simulink library "xblocks_library_downconverter"  (Simulink 7.6)
settings: Solver=ode45  SolverMode=SingleTasking  StartTime=0.0  StopTime=10.0  RelTol=1e-3
libraries: xbsIndex_r4 x104
settings Model: Creator=mdexter  LastModifiedBy=chenhong

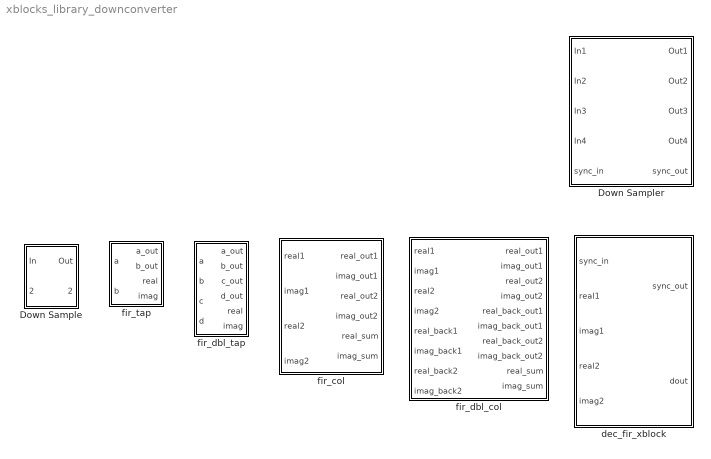
== system xblocks_library_downconverter ==
  Down Sample : Subsystem  mask(Down Sample){dec_rate=4, input_clk_period=1, input_period=2, xilinx=off, ext_en=off}
      mask prompts: dec_rate "Rate Change"; input_clk_period "Actual Input Clock Period"; input_period "Effective Input Sampling Period"; xilinx "Use Xilinx Down Sample?"; ext_en "External enable port?"
      mask help: Down Sample by using a periodically enabled register
      mask init:
      | config.source=str2func('downsample_init_xblock');
      | config.depend=get_dependlist('downsample');
      | config.toplevel=gcb;
      | set_param(gcb,'LinkStatus','inactive');
      | xBlock(config, {config.toplevel,...
      |     'dec_rate', dec_rate, ...
      |     'input_clk_period', input_clk_period, ...
      |     'input_period', input_period, ...
      |     'xilinx', xilinx, ...
      |     'ext_en', ext_en});
      settings: AttributesFormatString=|
      | Rate change: 4
      | clock(actualy/effective): 1/2
  Down Sampler : Subsystem  mask(Parallel Downconverter (xBlock)){n_inputs=4, dec_rate=3, xilinx=off, input_clk_rate=0}
      mask prompts: n_inputs "number of inputs"; dec_rate "Decimation rate"; xilinx "Use Xilinx version of Down Sample?"; input_clk_rate "Input Clock Rate"
      mask help: Parallely downconvert.
      mask init:
      | config.source=str2func('parallel_downsampler_init_xblock');
      | config.depend=get_dependlist('parallel_downsampler');
      | config.toplevel=gcb;
      | set_param(gcb,'LinkStatus','inactive');
      | xBlock(config, {config.toplevel,...
      |     'n_inputs', n_inputs, ...
      |     'dec_rate', dec_rate, ...
      |     'xilinx', xilinx, ...
      |     'input_clk_rate', input_clk_rate});
      settings: AttributesFormatString=Decimation Rate = 3
  dec_fir_xblock : Subsystem  mask(dec_fir (xBlock)){n_inputs=2, coeff=[1 2 3 4], n_bits=4, quantization=Truncate, add_latency=1, mult_latency=2, coeff_bit_width=25, coeff_bin_pt=24, adder_tree_hdl=off}
      mask prompts: n_inputs "Number of Parallel Streams"; coeff "Coefficients"; n_bits "Bit Width Out"; quantization "Quantization Behavior"; add_latency "Add Latency"; mult_latency "Mult Latency"; coeff_bit_width "Coefficient bit width"; coeff_bin_pt "Coefficient binary point"; adder_tree_hdl "Implement first stage of adder trees after multiplication as behavioural HDL"
      mask help:
      | FIR filter which can handle multiple time samples in parallel and decimates down to 1 time sample.  If coefficients are symmetric, will automatically fold before multiplying.
      | (xBlock version)
      mask init:
      | config.source=str2func('dec_fir_init_xblock');
      | config.toplevel=gcb;
      | config.depend = get_dependlist('dec_fir');
      | set_param(gcb,'LinkStatus','inactive');
      | xBlock(config, ...
      |         {config.toplevel,n_inputs,coeff,n_bits,quantization,add_latency,...
      |          mult_latency, coeff_bit_width,coeff_bin_pt,adder_tree_hdl});
      settings: AttributesFormatString=|
      | 4 taps
      | 4_3 r/i
      mask StyleString: edit,edit,edit,popup(Truncate|Round  (unbiased: +/- Inf)|Round  (unbiased: Even Values)),edit,edit,edit,edit,checkbox
      mask CallbackString:
      | coeff = (get_param(gcb,'coeff'));
      | n_inputs = (get_param(gcb,'n_inputs'));
      | if ~isempty(coeff) && ~isempty(n_inputs)
      |     coeff = eval(coeff);
      |     n_inputs = eval(n_inputs);
      |     coeff_round = round(coeff*1e16)*1e-16;
      |     if mod(length(coeff)/n_inputs,1) ~=0
      |         errordlg('The number of coefficients must be integer multiples of the number of inputs');
      |         set_param(gcb,'n_inputs','');
      |     end
      |     num_fir_col = length(coeff)/n_inputs;
      |     if coeff_round(1:int32(length(coeff)/2)) == coeff_round(length(coeff):-1:int32(length(coeff)/2)+1)
      |         num_fir_col = num_fir_col / 2;
      |     end
      |     if num_fir_col <= 0
      |         errordlg(['error: the number of column must be a positive integer. num_fir_col = ', num2str(num_fir_col)]);
      |         set_param(gcb,'n_inputs','');
      |     end
      | end
      | |coeff = (get_param(gcb,'coeff'));
      | n_inputs = (get_param(gcb,'n_inputs'));
      | if ~isempty(coeff) && ~isempty(n_inputs)
      |     coeff = eval(coeff);
      |     n_inputs = eval(n_inputs);
      |     coeff_round = round(coeff*1e16)*1e-16;
      |     if mod(length(coeff)/n_inputs,1) ~=0
      |         errordlg('The number of coefficients must be integer multiples of the number of inputs');
      |         set_param(gcb,'coeff','');
      |     end
      |     num_fir_col = length(coeff)/n_inputs;
      |     if coeff_round(1:int32(length(coeff)/2)) == coeff_round(length(coeff):-1:int32(length(coeff)/2)+1)
      |         num_fir_col = num_fir_col / 2;
      |     end
      |     if num_fir_col <= 0
      |         errordlg(['error: the number of column must be a positive integer. num_fir_col = ', num2str(num_fir_col)]);
      |         set_param(gcb,'coeff','');
      |     end
      | end
      | |||||||
  fir_col : Subsystem  mask(fir_col){n_inputs=2, coeff=[2 3], add_latency=1, mult_latency=2, coeff_bit_width=25, coeff_bin_pt=24, adder_tree_hdl=off}
      mask prompts: n_inputs "Inputs"; coeff "Coefficients"; add_latency "Add latency"; mult_latency "Mult Latency"; coeff_bit_width "Coefficient bit width"; coeff_bin_pt "Coefficient binary point"; adder_tree_hdl "Implement first stage of adder trees on output as behavioural HDL"
      mask help: (xBlock version)
      mask init:
      | config.source = str2func('fir_col_init_xblock');
      | config.toplevel = gcb;
      | config.depend = get_dependlist('fir_col');
      | set_param(gcb,'LinkStatus','inactive');
      | xBlock(config, {config.toplevel, ...
      |     n_inputs,...
      |     coeff, ...
      |     add_latency, ...
      |     mult_latency, ...
      |     coeff_bit_width, ...
      |     coeff_bin_pt, ...
      |     adder_tree_hdl});
      mask Help: eval('xlWeb(''http://casper.berkeley.edu/wiki/Fir_col'')')
  fir_dbl_col : Subsystem  mask(fir_dbl_col){n_inputs=2, coeff=[0.1 0.2 0.3 0.4], add_latency=1, mult_latency=2, coeff_bit_width=25, coeff_bin_pt=24, adder_tree_hdl=off}
      mask prompts: n_inputs "Inputs"; coeff "Coefficients"; add_latency "Add latency"; mult_latency "Mult Latency"; coeff_bit_width "Coefficient bit width"; coeff_bin_pt "Coefficient binary point"; adder_tree_hdl "Implement first stage of adder trees on output as behavioural HDL"
      mask help: (xBlock version)
      mask init:
      | config.source = str2func('fir_dbl_col_init_xblock');
      | config.toplevel = gcb;
      | config.depend = get_dependlist('fir_dbl_col');
      | set_param(gcb,'LinkStatus','inactive');
      | xBlock(config, {config.toplevel, ...
      |      n_inputs, ...
      |      coeff, ...
      |      add_latency, ...
      |      mult_latency, ...
      |      coeff_bit_width, ...
      |      coeff_bin_pt,  ...
      |      adder_tree_hdl});
      mask Help: eval('xlWeb(''http://casper.berkeley.edu/wiki/Fir_dbl_col'')')
  fir_dbl_tap : Subsystem  mask(fir_dbl_tap){factor=0.073384, add_latency=1, mult_latency=2, coeff_bit_width=18, coeff_bin_pt=17}
      mask prompts: add_latency "Add latency"; mult_latency "Mult latency"; coeff_bit_width "Coefficient bit width"; coeff_bin_pt "Coefficient binary point"
      mask help: (xBlock version)
      mask init:
      | config.source = str2func('fir_dbl_tap_init_xblock');
      | config.toplevel = gcb;
      | config.depend = get_dependlist('fir_dbl_tap');
      | set_param(gcb,'LinkStatus','inactive');
      | xBlock(config, {config.toplevel, ...
      |     factor, ...
      |     add_latency, ...
      |     mult_latency, ...
      |     coeff_bit_width, ...
      |     coeff_bin_pt});
      mask Help: eval('xlWeb(''http://casper.berkeley.edu/wiki/Fir_dbl_tap'')')
  fir_tap : Subsystem  mask(fir_tap){factor=1, latency=2, coeff_bit_width=25, coeff_bin_pt=24}
      mask prompts: latency "Mult latency"; coeff_bit_width "Coefficient bit width"; coeff_bin_pt "Coefficient binary point"
      mask help:
      | Multiplies input data with factor specified.
      | (xBlock version)
      mask init:
      | config.source = str2func('fir_tap_init_xblock');
      | config.toplevel = gcb;
      | config.depend = get_dependlist('fir_tap');
      | set_param(gcb,'LinkStatus','inactive');
      | xBlock(config,{config.toplevel, ...
      |     factor, ...
      |     latency, ...
      |     coeff_bit_width, ...
      |     coeff_bin_pt});
      mask Help: eval('xlWeb(''http://casper.berkeley.edu/wiki/Fir_tap'')')

== system xblocks_library_downconverter/Down Sample ==
  In : Inport
  sync_in : Inport  Port=2
  Register : xbsIndex_r4/Register  init=0  rst=off  en=on  dbl_ovrd=off  block_type=register
  en_gen : Subsystem
      settings: AttributesFormatString=|
      | hold period: 8
      | explicit clk period:on , input clk period:1
  sync_delay : xbsIndex_r4/Delay  rst=off  infoeditControl=Selection of Reset will increase slice count due to use of real FFs and instead of SRLs  en=off  latency=1  dbl_ovrd=off  reg_retiming=off  block_type=delay
  Out : Outport
  sync_out : Outport  Port=2
  wires:
  sync_in/1 -> sync_delay/1, en_gen/1(sync_in)
  sync_delay/1 -> sync_out/1
  Register/1 -> Out/1
  en_gen/1(en_out) -> Register/2  "en"
  In/1 -> Register/1

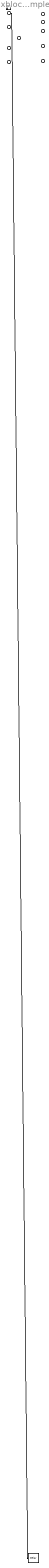
== system xblocks_library_downconverter/Down Sampler ==
  In1 : Inport
  In2 : Inport  Port=2
  In3 : Inport  Port=3
  In4 : Inport  Port=4
  sync_in : Inport  Port=5
  Down_sample1 : Subsystem
  delay1 : xbsIndex_r4/Delay  rst=off  infoeditControl=Selection of Reset will increase slice count due to use of real FFs and instead of SRLs  en=off  latency=2  dbl_ovrd=off  reg_retiming=off  block_type=delay
  Out1 : Outport
  Out2 : Outport  Port=2
  Out3 : Outport  Port=3
  Out4 : Outport  Port=4
  sync_out : Outport  Port=5
  wires:
  In1/1 -> delay1/1

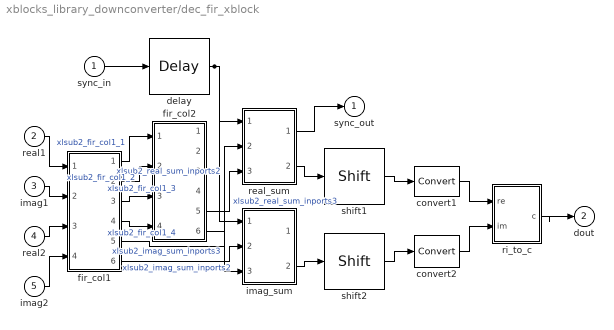
== system xblocks_library_downconverter/dec_fir_xblock ==
  sync_in : Inport
  real1 : Inport  Port=2
  imag1 : Inport  Port=3
  real2 : Inport  Port=4
  imag2 : Inport  Port=5
  convert1 : xbsIndex_r4/Convert  gui_display_data_type=Fixed-point  arith_type="Signed  (2's comp)"  n_bits=4  bin_pt=3  float_type=Single  exp_bits=8  fraction_bits=24  quantization=Truncate  overflow=Wrap  en=off  latency=1  dbl_ovrd=off  pipeline=off  block_type=convert
  convert2 : xbsIndex_r4/Convert  gui_display_data_type=Fixed-point  arith_type="Signed  (2's comp)"  n_bits=4  bin_pt=3  float_type=Single  exp_bits=8  fraction_bits=24  quantization=Truncate  overflow=Wrap  en=off  latency=1  dbl_ovrd=off  pipeline=off  block_type=convert
  delay : xbsIndex_r4/Delay  rst=off  infoeditControl=Selection of Reset will increase slice count due to use of real FFs and instead of SRLs  en=off  latency=4  dbl_ovrd=off  reg_retiming=off  block_type=delay
  fir_col1 : Subsystem
  fir_col2 : Subsystem
  imag_sum : Subsystem
      settings: AttributesFormatString=latency 1
  real_sum : Subsystem
      settings: AttributesFormatString=latency 1
  ri_to_c : Subsystem
  shift1 : xbsIndex_r4/Shift  shift_dir=Left  shift_bits=1  en=off  latency=0  precision=Full  arith_type="Signed  (2's comp)"  n_bits=16  bin_pt=14  quantization=Truncate  overflow=Wrap  dbl_ovrd=off  block_type=shift
  shift2 : xbsIndex_r4/Shift  shift_dir=Left  shift_bits=1  en=off  latency=0  precision=Full  arith_type="Signed  (2's comp)"  n_bits=16  bin_pt=14  quantization=Truncate  overflow=Wrap  dbl_ovrd=off  block_type=shift
  sync_out : Outport
  dout : Outport  Port=2
  wires:
  delay/1 -> real_sum/1(sync), imag_sum/1(sync)
  shift2/1 -> convert2/1
  imag_sum/2(dout) -> shift2/1
  shift1/1 -> convert1/1
  real_sum/2(dout) -> shift1/1
  ri_to_c/1(c) -> dout/1
  convert2/1 -> ri_to_c/2(im)
  convert1/1 -> ri_to_c/1(re)
  real_sum/1(sync_out) -> sync_out/1
  fir_col2/5(real_sum) -> real_sum/3(din2)  "xlsub2_real_sum_inports3"
  fir_col1/5(real_sum) -> real_sum/2(din1)  "xlsub2_real_sum_inports2"
  fir_col2/6(imag_sum) -> imag_sum/3(din2)  "xlsub2_imag_sum_inports3"
  fir_col1/6(imag_sum) -> imag_sum/2(din1)  "xlsub2_imag_sum_inports2"
  fir_col1/4(imag_out2) -> fir_col2/4(imag2)  "xlsub2_fir_col1_4"
  fir_col1/3(real_out2) -> fir_col2/3(real2)  "xlsub2_fir_col1_3"
  fir_col1/2(imag_out1) -> fir_col2/2(imag1)  "xlsub2_fir_col1_2"
  fir_col1/1(real_out1) -> fir_col2/1(real1)  "xlsub2_fir_col1_1"
  imag2/1 -> fir_col1/4(imag2)
  real2/1 -> fir_col1/3(real2)
  imag1/1 -> fir_col1/2(imag1)
  real1/1 -> fir_col1/1(real1)
  sync_in/1 -> delay/1

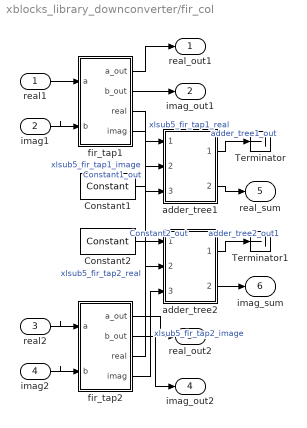
== system xblocks_library_downconverter/fir_col ==
  real1 : Inport
  imag1 : Inport  Port=2
  real2 : Inport  Port=3
  imag2 : Inport  Port=4
  Constant1 : xbsIndex_r4/Constant  arith_type=Signed (2's comp)  const=1  n_bits=16  bin_pt=14  explicit_period=on  period=1  equ=P=C  opselect=C  inp2=PCIN>>17  opr=+  inp1=P  carry=CIN  dbl_ovrd=off  block_type=constant
      settings: block_version=11.4
  Constant2 : xbsIndex_r4/Constant  arith_type=Signed (2's comp)  const=1  n_bits=16  bin_pt=14  explicit_period=on  period=1  equ=P=C  opselect=C  inp2=PCIN>>17  opr=+  inp1=P  carry=CIN  dbl_ovrd=off  block_type=constant
      settings: block_version=11.4
  Terminator : Terminator
  Terminator1 : Terminator
  adder_tree1 : Subsystem
      settings: AttributesFormatString=latency 1
  adder_tree2 : Subsystem
      settings: AttributesFormatString=latency 1
  fir_tap1 : Subsystem
  fir_tap2 : Subsystem
  real_out1 : Outport
  imag_out1 : Outport  Port=2
  real_out2 : Outport  Port=3
  imag_out2 : Outport  Port=4
  real_sum : Outport  Port=5
  imag_sum : Outport  Port=6
  wires:
  adder_tree2/1(sync_out) -> Terminator1/1  "adder_tree2_out1"
  adder_tree1/1(sync_out) -> Terminator/1  "adder_tree1_out"
  adder_tree2/2(dout) -> imag_sum/1
  fir_tap2/4(imag) -> adder_tree2/3(din2)  "xlsub5_fir_tap2_image"
  fir_tap1/4(imag) -> adder_tree2/2(din1)  "xlsub5_fir_tap1_image"
  Constant2/1 -> adder_tree2/1(sync)  "Constant2_out"
  adder_tree1/2(dout) -> real_sum/1
  fir_tap2/3(real) -> adder_tree1/3(din2)  "xlsub5_fir_tap2_real"
  fir_tap1/3(real) -> adder_tree1/2(din1)  "xlsub5_fir_tap1_real"
  Constant1/1 -> adder_tree1/1(sync)  "Constant1_out"
  fir_tap2/2(b_out) -> imag_out2/1
  fir_tap2/1(a_out) -> real_out2/1
  imag2/1 -> fir_tap2/2(b)
  real2/1 -> fir_tap2/1(a)
  fir_tap1/2(b_out) -> imag_out1/1
  fir_tap1/1(a_out) -> real_out1/1
  imag1/1 -> fir_tap1/2(b)
  real1/1 -> fir_tap1/1(a)

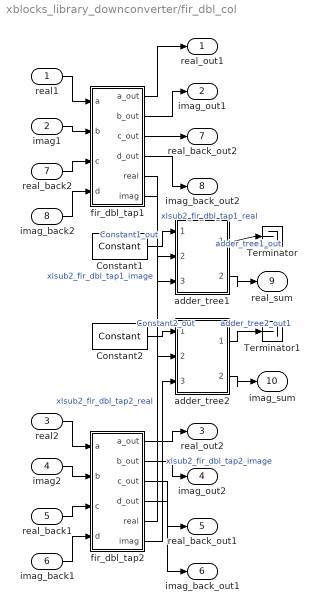
== system xblocks_library_downconverter/fir_dbl_col ==
  real1 : Inport
  imag1 : Inport  Port=2
  real2 : Inport  Port=3
  imag2 : Inport  Port=4
  real_back1 : Inport  Port=5
  imag_back1 : Inport  Port=6
  real_back2 : Inport  Port=7
  imag_back2 : Inport  Port=8
  Constant1 : xbsIndex_r4/Constant  arith_type=Signed (2's comp)  const=1  n_bits=16  bin_pt=14  explicit_period=on  period=1  equ=P=C  opselect=C  inp2=PCIN>>17  opr=+  inp1=P  carry=CIN  dbl_ovrd=off  block_type=constant
      settings: block_version=11.4
  Constant2 : xbsIndex_r4/Constant  arith_type=Signed (2's comp)  const=1  n_bits=16  bin_pt=14  explicit_period=on  period=1  equ=P=C  opselect=C  inp2=PCIN>>17  opr=+  inp1=P  carry=CIN  dbl_ovrd=off  block_type=constant
      settings: block_version=11.4
  Terminator : Terminator
  Terminator1 : Terminator
  adder_tree1 : Subsystem
      settings: AttributesFormatString=latency 1
  adder_tree2 : Subsystem
      settings: AttributesFormatString=latency 1
  fir_dbl_tap1 : Subsystem
  fir_dbl_tap2 : Subsystem
  real_out1 : Outport
  imag_out1 : Outport  Port=2
  real_out2 : Outport  Port=3
  imag_out2 : Outport  Port=4
  real_back_out1 : Outport  Port=5
  imag_back_out1 : Outport  Port=6
  real_back_out2 : Outport  Port=7
  imag_back_out2 : Outport  Port=8
  real_sum : Outport  Port=9
  imag_sum : Outport  Port=10
  wires:
  adder_tree2/1(sync_out) -> Terminator1/1  "adder_tree2_out1"
  adder_tree1/1(sync_out) -> Terminator/1  "adder_tree1_out"
  adder_tree2/2(dout) -> imag_sum/1
  fir_dbl_tap2/6(imag) -> adder_tree2/3(din2)  "xlsub2_fir_dbl_tap2_image"
  fir_dbl_tap1/6(imag) -> adder_tree2/2(din1)  "xlsub2_fir_dbl_tap1_image"
  Constant2/1 -> adder_tree2/1(sync)  "Constant2_out"
  adder_tree1/2(dout) -> real_sum/1
  fir_dbl_tap2/5(real) -> adder_tree1/3(din2)  "xlsub2_fir_dbl_tap2_real"
  fir_dbl_tap1/5(real) -> adder_tree1/2(din1)  "xlsub2_fir_dbl_tap1_real"
  Constant1/1 -> adder_tree1/1(sync)  "Constant1_out"
  fir_dbl_tap2/4(d_out) -> imag_back_out1/1
  fir_dbl_tap2/3(c_out) -> real_back_out1/1
  fir_dbl_tap2/2(b_out) -> imag_out2/1
  fir_dbl_tap2/1(a_out) -> real_out2/1
  imag_back1/1 -> fir_dbl_tap2/4(d)
  real_back1/1 -> fir_dbl_tap2/3(c)
  imag2/1 -> fir_dbl_tap2/2(b)
  real2/1 -> fir_dbl_tap2/1(a)
  fir_dbl_tap1/4(d_out) -> imag_back_out2/1
  fir_dbl_tap1/3(c_out) -> real_back_out2/1
  fir_dbl_tap1/2(b_out) -> imag_out1/1
  fir_dbl_tap1/1(a_out) -> real_out1/1
  imag_back2/1 -> fir_dbl_tap1/4(d)
  real_back2/1 -> fir_dbl_tap1/3(c)
  imag1/1 -> fir_dbl_tap1/2(b)
  real1/1 -> fir_dbl_tap1/1(a)

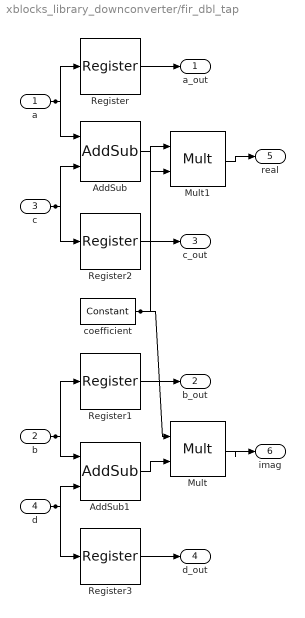
== system xblocks_library_downconverter/fir_dbl_tap ==
  a : Inport
  b : Inport  Port=2
  c : Inport  Port=3
  d : Inport  Port=4
  AddSub : xbsIndex_r4/AddSub  mode=Addition  use_carryin=off  use_carryout=off  en=off  latency=1  precision=Full  arith_type="Signed  (2's comp)"  n_bits=18  bin_pt=16  quantization=Truncate  overflow=Wrap  dbl_ovrd=off  use_behavioral_HDL=on  hw_selection=Fabric  pipelined=off  use_rpm=on  block_type=addsub
  AddSub1 : xbsIndex_r4/AddSub  mode=Addition  use_carryin=off  use_carryout=off  en=off  latency=1  precision=Full  arith_type="Signed  (2's comp)"  n_bits=18  bin_pt=16  quantization=Truncate  overflow=Wrap  dbl_ovrd=off  use_behavioral_HDL=on  hw_selection=Fabric  pipelined=off  use_rpm=on  block_type=addsub
  Mult : xbsIndex_r4/Mult  precision=Full  arith_type="Signed  (2's comp)"  n_bits=18  bin_pt=17  quantization=Truncate  overflow=Wrap  en=off  latency=2  dbl_ovrd=off  use_behavioral_HDL=on  opt=Speed  use_embedded=on  optimum_pipeline=off  pipeline=on  use_rpm=off  placement_style=Rectangular shape  block_type=mult
      settings: block_version=11.4
  Mult1 : xbsIndex_r4/Mult  precision=Full  arith_type="Signed  (2's comp)"  n_bits=18  bin_pt=17  quantization=Truncate  overflow=Wrap  en=off  latency=2  dbl_ovrd=off  use_behavioral_HDL=on  opt=Speed  use_embedded=on  optimum_pipeline=off  pipeline=on  use_rpm=off  placement_style=Rectangular shape  block_type=mult
      settings: block_version=11.4
  Register{,1..3} (4 alike) : xbsIndex_r4/Register  init=0  rst=off  en=off  dbl_ovrd=off  block_type=register
      settings: block_version=11.4
  coefficient : xbsIndex_r4/Constant  arith_type=Signed (2's comp)  const=0.073384  n_bits=18  bin_pt=17  explicit_period=on  period=1  equ=P=C  opselect=C  inp2=PCIN>>17  opr=+  inp1=P  carry=CIN  dbl_ovrd=off  block_type=constant
      settings: block_version=11.4
  a_out : Outport
  b_out : Outport  Port=2
  c_out : Outport  Port=3
  d_out : Outport  Port=4
  real : Outport  Port=5
  imag : Outport  Port=6
  wires:
  a/1 -> Register/1, AddSub/1
  c/1 -> Register2/1, AddSub/2
  b/1 -> Register1/1, AddSub1/1
  d/1 -> Register3/1, AddSub1/2
  coefficient/1 -> Mult1/1, Mult/1
  Register3/1 -> d_out/1
  Register2/1 -> c_out/1
  Register1/1 -> b_out/1
  Register/1 -> a_out/1
  Mult1/1 -> real/1
  AddSub/1 -> Mult1/2
  Mult/1 -> imag/1
  AddSub1/1 -> Mult/2

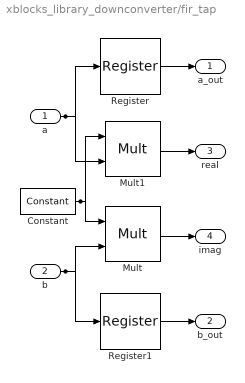
== system xblocks_library_downconverter/fir_tap ==
  a : Inport
  b : Inport  Port=2
  Constant : xbsIndex_r4/Constant  const=1  gui_display_data_type=Fixed-point  arith_type=Signed (2's comp)  n_bits=25  bin_pt=24  preci_type=Single  exp_width=8  frac_width=24  explicit_period=on  period=1  equ=P=C  opselect=C  inp2=PCIN>>17  opr=+  inp1=P  carry=CIN  dbl_ovrd=off  block_type=constant
  Mult : xbsIndex_r4/Mult  precision=Full  arith_type="Signed  (2's comp)"  n_bits=18  bin_pt=17  quantization=Truncate  overflow=Wrap  en=off  latency=2  dbl_ovrd=off  use_behavioral_HDL=on  opt=Speed  use_embedded=on  optimum_pipeline=off  pipeline=on  use_rpm=off  placement_style=Rectangular shape  block_type=mult
  Mult1 : xbsIndex_r4/Mult  precision=Full  arith_type="Signed  (2's comp)"  n_bits=18  bin_pt=17  quantization=Truncate  overflow=Wrap  en=off  latency=2  dbl_ovrd=off  use_behavioral_HDL=on  opt=Speed  use_embedded=on  optimum_pipeline=off  pipeline=on  use_rpm=off  placement_style=Rectangular shape  block_type=mult
  Register : xbsIndex_r4/Register  init=0  rst=off  en=off  dbl_ovrd=off  block_type=register
  Register1 : xbsIndex_r4/Register  init=0  rst=off  en=off  dbl_ovrd=off  block_type=register
  a_out : Outport
  b_out : Outport  Port=2
  real : Outport  Port=3
  imag : Outport  Port=4
  wires:
  Constant/1 -> Mult1/1, Mult/1
  b/1 -> Register1/1, Mult/2
  a/1 -> Register/1, Mult1/2
  Register1/1 -> b_out/1
  Register/1 -> a_out/1
  Mult1/1 -> real/1
  Mult/1 -> imag/1

== system xblocks_library_downconverter/Down Sample/en_gen ==
  sync_in : Inport
  Constant : xbsIndex_r4/Constant  const=0  gui_display_data_type=Fixed-point  arith_type=Signed (2's comp)  n_bits=16  bin_pt=14  preci_type=Single  exp_width=8  frac_width=24  explicit_period=off  period=1  equ=P=C  opselect=C  inp2=PCIN>>17  opr=+  inp1=P  carry=CIN  dbl_ovrd=off  block_type=constant
  Counter1 : xbsIndex_r4/Counter  cnt_type=Count Limited  cnt_to=0  operation=Down  start_count=7  cnt_by_val=1  arith_type=Unsigned  n_bits=3  bin_pt=0  load_pin=off  rst=on  en=off  explicit_period=on  period=1  dbl_ovrd=off  use_behavioral_HDL=off  implementation=Fabric  block_type=counter
  Relational : xbsIndex_r4/Relational  mode=a=b  en=off  latency=1  dbl_ovrd=off  block_type=relational
  en_out : Outport
  wires:
  Relational/1 -> en_out/1
  Constant/1 -> Relational/2  "xlsub1_Constant_out1"
  Counter1/1 -> Relational/1  "xlsub1_Counter1_out1"
  sync_in/1 -> Counter1/1

== system xblocks_library_downconverter/Down Sampler/Down_sample1 ==
  In : Inport
  sync_in : Inport  Port=2
  Out : Outport
  sync_out : Outport  Port=2

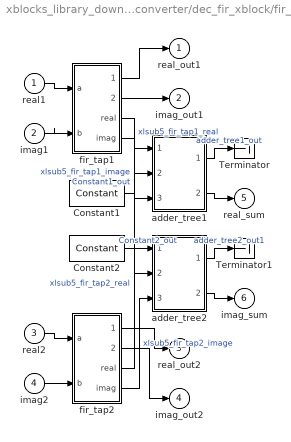
== system xblocks_library_downconverter/dec_fir_xblock/fir_col1 ==
  real1 : Inport
  imag1 : Inport  Port=2
  real2 : Inport  Port=3
  imag2 : Inport  Port=4
  Constant1 : xbsIndex_r4/Constant  const=1  gui_display_data_type=Fixed-point  arith_type=Signed (2's comp)  n_bits=16  bin_pt=14  preci_type=Single  exp_width=8  frac_width=24  explicit_period=on  period=1  equ=P=C  opselect=C  inp2=PCIN>>17  opr=+  inp1=P  carry=CIN  dbl_ovrd=off  block_type=constant
  Constant2 : xbsIndex_r4/Constant  const=1  gui_display_data_type=Fixed-point  arith_type=Signed (2's comp)  n_bits=16  bin_pt=14  preci_type=Single  exp_width=8  frac_width=24  explicit_period=on  period=1  equ=P=C  opselect=C  inp2=PCIN>>17  opr=+  inp1=P  carry=CIN  dbl_ovrd=off  block_type=constant
  Terminator : Terminator
  Terminator1 : Terminator
  adder_tree1 : Subsystem
      settings: AttributesFormatString=latency 2
  adder_tree2 : Subsystem
      settings: AttributesFormatString=latency 2
  fir_tap1 : Subsystem
  fir_tap2 : Subsystem
  real_out1 : Outport
  imag_out1 : Outport  Port=2
  real_out2 : Outport  Port=3
  imag_out2 : Outport  Port=4
  real_sum : Outport  Port=5
  imag_sum : Outport  Port=6
  wires:
  adder_tree2/1(sync_out) -> Terminator1/1  "adder_tree2_out1"
  adder_tree1/1(sync_out) -> Terminator/1  "adder_tree1_out"
  adder_tree2/2(dout) -> imag_sum/1
  fir_tap2/4(imag) -> adder_tree2/3(din2)  "xlsub5_fir_tap2_image"
  fir_tap1/4(imag) -> adder_tree2/2(din1)  "xlsub5_fir_tap1_image"
  Constant2/1 -> adder_tree2/1(sync)  "Constant2_out"
  adder_tree1/2(dout) -> real_sum/1
  fir_tap2/3(real) -> adder_tree1/3(din2)  "xlsub5_fir_tap2_real"
  fir_tap1/3(real) -> adder_tree1/2(din1)  "xlsub5_fir_tap1_real"
  Constant1/1 -> adder_tree1/1(sync)  "Constant1_out"
  fir_tap2/2(b_out) -> imag_out2/1
  fir_tap2/1(a_out) -> real_out2/1
  imag2/1 -> fir_tap2/2(b)
  real2/1 -> fir_tap2/1(a)
  fir_tap1/2(b_out) -> imag_out1/1
  fir_tap1/1(a_out) -> real_out1/1
  imag1/1 -> fir_tap1/2(b)
  real1/1 -> fir_tap1/1(a)

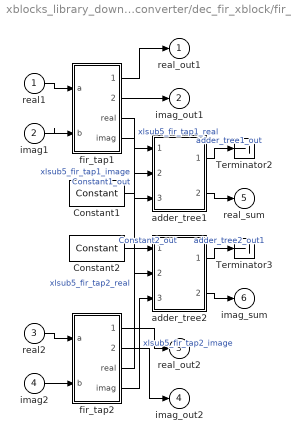
== system xblocks_library_downconverter/dec_fir_xblock/fir_col2 ==
  real1 : Inport
  imag1 : Inport  Port=2
  real2 : Inport  Port=3
  imag2 : Inport  Port=4
  Constant1 : xbsIndex_r4/Constant  const=1  gui_display_data_type=Fixed-point  arith_type=Signed (2's comp)  n_bits=16  bin_pt=14  preci_type=Single  exp_width=8  frac_width=24  explicit_period=on  period=1  equ=P=C  opselect=C  inp2=PCIN>>17  opr=+  inp1=P  carry=CIN  dbl_ovrd=off  block_type=constant
  Constant2 : xbsIndex_r4/Constant  const=1  gui_display_data_type=Fixed-point  arith_type=Signed (2's comp)  n_bits=16  bin_pt=14  preci_type=Single  exp_width=8  frac_width=24  explicit_period=on  period=1  equ=P=C  opselect=C  inp2=PCIN>>17  opr=+  inp1=P  carry=CIN  dbl_ovrd=off  block_type=constant
  Terminator2 : Terminator
  Terminator3 : Terminator
  adder_tree1 : Subsystem
      settings: AttributesFormatString=latency 2
  adder_tree2 : Subsystem
      settings: AttributesFormatString=latency 2
  fir_tap1 : Subsystem
  fir_tap2 : Subsystem
  real_out1 : Outport
  imag_out1 : Outport  Port=2
  real_out2 : Outport  Port=3
  imag_out2 : Outport  Port=4
  real_sum : Outport  Port=5
  imag_sum : Outport  Port=6
  wires:
  adder_tree2/1(sync_out) -> Terminator3/1  "adder_tree2_out1"
  adder_tree1/1(sync_out) -> Terminator2/1  "adder_tree1_out"
  adder_tree2/2(dout) -> imag_sum/1
  fir_tap2/4(imag) -> adder_tree2/3(din2)  "xlsub5_fir_tap2_image"
  fir_tap1/4(imag) -> adder_tree2/2(din1)  "xlsub5_fir_tap1_image"
  Constant2/1 -> adder_tree2/1(sync)  "Constant2_out"
  adder_tree1/2(dout) -> real_sum/1
  fir_tap2/3(real) -> adder_tree1/3(din2)  "xlsub5_fir_tap2_real"
  fir_tap1/3(real) -> adder_tree1/2(din1)  "xlsub5_fir_tap1_real"
  Constant1/1 -> adder_tree1/1(sync)  "Constant1_out"
  fir_tap2/2(b_out) -> imag_out2/1
  fir_tap2/1(a_out) -> real_out2/1
  imag2/1 -> fir_tap2/2(b)
  real2/1 -> fir_tap2/1(a)
  fir_tap1/2(b_out) -> imag_out1/1
  fir_tap1/1(a_out) -> real_out1/1
  imag1/1 -> fir_tap1/2(b)
  real1/1 -> fir_tap1/1(a)

== system xblocks_library_downconverter/dec_fir_xblock/imag_sum ==
  sync : Inport
  din1 : Inport  Port=2
  din2 : Inport  Port=3
  addr1 : xbsIndex_r4/AddSub  mode=Addition  use_carryin=off  use_carryout=off  en=off  latency=1  precision=Full  arith_type=Unsigned  n_bits=16  bin_pt=14  quantization=Truncate  overflow=Wrap  dbl_ovrd=off  use_behavioral_HDL=off  hw_selection=Fabric  pipelined=on  use_rpm=on  block_type=addsub
  sync_delay : xbsIndex_r4/Delay  rst=off  infoeditControl=Selection of Reset will increase slice count due to use of real FFs and instead of SRLs  en=off  latency=1  dbl_ovrd=off  reg_retiming=on  block_type=delay
  sync_out : Outport
  dout : Outport  Port=2
  wires:
  addr1/1 -> dout/1  "adder_outs1_1"
  din2/1 -> addr1/2
  din1/1 -> addr1/1
  sync_delay/1 -> sync_out/1
  sync/1 -> sync_delay/1

== system xblocks_library_downconverter/dec_fir_xblock/real_sum ==
  sync : Inport
  din1 : Inport  Port=2
  din2 : Inport  Port=3
  addr1 : xbsIndex_r4/AddSub  mode=Addition  use_carryin=off  use_carryout=off  en=off  latency=1  precision=Full  arith_type=Unsigned  n_bits=16  bin_pt=14  quantization=Truncate  overflow=Wrap  dbl_ovrd=off  use_behavioral_HDL=off  hw_selection=Fabric  pipelined=on  use_rpm=on  block_type=addsub
  sync_delay : xbsIndex_r4/Delay  rst=off  infoeditControl=Selection of Reset will increase slice count due to use of real FFs and instead of SRLs  en=off  latency=1  dbl_ovrd=off  reg_retiming=on  block_type=delay
  sync_out : Outport
  dout : Outport  Port=2
  wires:
  addr1/1 -> dout/1  "adder_outs1_1"
  din2/1 -> addr1/2
  din1/1 -> addr1/1
  sync_delay/1 -> sync_out/1
  sync/1 -> sync_delay/1

== system xblocks_library_downconverter/dec_fir_xblock/ri_to_c ==
  re : Inport
  im : Inport  Port=2
  concat : xbsIndex_r4/Concat  num_inputs=2  dbl_ovrd=off  block_type=concat
  force_im : xbsIndex_r4/Reinterpret  force_arith_type=on  arith_type=Unsigned  force_bin_pt=on  bin_pt=0  block_type=reinterpret
  force_re : xbsIndex_r4/Reinterpret  force_arith_type=on  arith_type=Unsigned  force_bin_pt=on  bin_pt=0  block_type=reinterpret
  c : Outport
  wires:
  force_re/1 -> concat/1
  re/1 -> force_re/1
  force_im/1 -> concat/2
  im/1 -> force_im/1
  concat/1 -> c/1

== system xblocks_library_downconverter/fir_col/adder_tree1 ==
  sync : Inport
  din1 : Inport  Port=2
  din2 : Inport  Port=3
  addr1 : xbsIndex_r4/AddSub  mode=Addition  use_carryin=off  use_carryout=off  en=off  latency=1  precision=Full  arith_type=Unsigned  n_bits=16  bin_pt=14  quantization=Truncate  overflow=Wrap  dbl_ovrd=off  use_behavioral_HDL=off  hw_selection=Fabric  pipelined=on  use_rpm=on  block_type=addsub
  sync_delay : xbsIndex_r4/Delay  en=off  latency=1  dbl_ovrd=off  reg_retiming=on  block_type=delay
      settings: block_version=11.4
  sync_out : Outport
  dout : Outport  Port=2
  wires:
  addr1/1 -> dout/1  "adder_outs1_1"
  din2/1 -> addr1/2
  din1/1 -> addr1/1
  sync_delay/1 -> sync_out/1
  sync/1 -> sync_delay/1

== system xblocks_library_downconverter/fir_col/adder_tree2 ==
  sync : Inport
  din1 : Inport  Port=2
  din2 : Inport  Port=3
  addr1 : xbsIndex_r4/AddSub  mode=Addition  use_carryin=off  use_carryout=off  en=off  latency=1  precision=Full  arith_type=Unsigned  n_bits=16  bin_pt=14  quantization=Truncate  overflow=Wrap  dbl_ovrd=off  use_behavioral_HDL=off  hw_selection=Fabric  pipelined=on  use_rpm=on  block_type=addsub
  sync_delay : xbsIndex_r4/Delay  en=off  latency=1  dbl_ovrd=off  reg_retiming=on  block_type=delay
      settings: block_version=11.4
  sync_out : Outport
  dout : Outport  Port=2
  wires:
  addr1/1 -> dout/1  "adder_outs1_1"
  din2/1 -> addr1/2
  din1/1 -> addr1/1
  sync_delay/1 -> sync_out/1
  sync/1 -> sync_delay/1

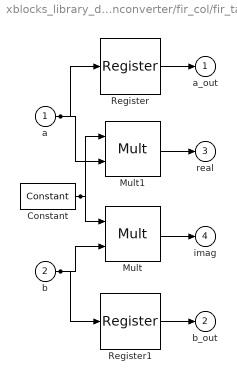
== system xblocks_library_downconverter/fir_col/fir_tap1 ==
  a : Inport
  b : Inport  Port=2
  Constant : xbsIndex_r4/Constant  arith_type=Signed (2's comp)  const=2  n_bits=25  bin_pt=24  explicit_period=on  period=1  equ=P=C  opselect=C  inp2=PCIN>>17  opr=+  inp1=P  carry=CIN  dbl_ovrd=off  block_type=constant
      settings: block_version=11.4
  Mult : xbsIndex_r4/Mult  precision=Full  arith_type="Signed  (2's comp)"  n_bits=18  bin_pt=17  quantization=Truncate  overflow=Wrap  en=off  latency=2  dbl_ovrd=off  use_behavioral_HDL=on  opt=Speed  use_embedded=on  optimum_pipeline=off  pipeline=on  use_rpm=off  placement_style=Rectangular shape  block_type=mult
      settings: block_version=11.4
  Mult1 : xbsIndex_r4/Mult  precision=Full  arith_type="Signed  (2's comp)"  n_bits=18  bin_pt=17  quantization=Truncate  overflow=Wrap  en=off  latency=2  dbl_ovrd=off  use_behavioral_HDL=on  opt=Speed  use_embedded=on  optimum_pipeline=off  pipeline=on  use_rpm=off  placement_style=Rectangular shape  block_type=mult
      settings: block_version=11.4
  Register : xbsIndex_r4/Register  init=0  rst=off  en=off  dbl_ovrd=off  block_type=register
      settings: block_version=11.4
  Register1 : xbsIndex_r4/Register  init=0  rst=off  en=off  dbl_ovrd=off  block_type=register
      settings: block_version=11.4
  a_out : Outport
  b_out : Outport  Port=2
  real : Outport  Port=3
  imag : Outport  Port=4
  wires:
  Constant/1 -> Mult1/1, Mult/1
  b/1 -> Register1/1, Mult/2
  a/1 -> Register/1, Mult1/2
  Register1/1 -> b_out/1
  Register/1 -> a_out/1
  Mult1/1 -> real/1
  Mult/1 -> imag/1

== system xblocks_library_downconverter/fir_col/fir_tap2 ==
  a : Inport
  b : Inport  Port=2
  Constant : xbsIndex_r4/Constant  arith_type=Signed (2's comp)  const=3  n_bits=25  bin_pt=24  explicit_period=on  period=1  equ=P=C  opselect=C  inp2=PCIN>>17  opr=+  inp1=P  carry=CIN  dbl_ovrd=off  block_type=constant
      settings: block_version=11.4
  Mult : xbsIndex_r4/Mult  precision=Full  arith_type="Signed  (2's comp)"  n_bits=18  bin_pt=17  quantization=Truncate  overflow=Wrap  en=off  latency=2  dbl_ovrd=off  use_behavioral_HDL=on  opt=Speed  use_embedded=on  optimum_pipeline=off  pipeline=on  use_rpm=off  placement_style=Rectangular shape  block_type=mult
      settings: block_version=11.4
  Mult1 : xbsIndex_r4/Mult  precision=Full  arith_type="Signed  (2's comp)"  n_bits=18  bin_pt=17  quantization=Truncate  overflow=Wrap  en=off  latency=2  dbl_ovrd=off  use_behavioral_HDL=on  opt=Speed  use_embedded=on  optimum_pipeline=off  pipeline=on  use_rpm=off  placement_style=Rectangular shape  block_type=mult
      settings: block_version=11.4
  Register : xbsIndex_r4/Register  init=0  rst=off  en=off  dbl_ovrd=off  block_type=register
      settings: block_version=11.4
  Register1 : xbsIndex_r4/Register  init=0  rst=off  en=off  dbl_ovrd=off  block_type=register
      settings: block_version=11.4
  a_out : Outport
  b_out : Outport  Port=2
  real : Outport  Port=3
  imag : Outport  Port=4
  wires:
  Constant/1 -> Mult1/1, Mult/1
  b/1 -> Register1/1, Mult/2
  a/1 -> Register/1, Mult1/2
  Register1/1 -> b_out/1
  Register/1 -> a_out/1
  Mult1/1 -> real/1
  Mult/1 -> imag/1

== system xblocks_library_downconverter/fir_dbl_col/adder_tree1 ==
  sync : Inport
  din1 : Inport  Port=2
  din2 : Inport  Port=3
  addr1 : xbsIndex_r4/AddSub  mode=Addition  use_carryin=off  use_carryout=off  en=off  latency=1  precision=Full  arith_type=Unsigned  n_bits=16  bin_pt=14  quantization=Truncate  overflow=Wrap  dbl_ovrd=off  use_behavioral_HDL=off  hw_selection=Fabric  pipelined=on  use_rpm=on  block_type=addsub
  sync_delay : xbsIndex_r4/Delay  en=off  latency=1  dbl_ovrd=off  reg_retiming=on  block_type=delay
      settings: block_version=11.4
  sync_out : Outport
  dout : Outport  Port=2
  wires:
  addr1/1 -> dout/1  "adder_outs1_1"
  din2/1 -> addr1/2
  din1/1 -> addr1/1
  sync_delay/1 -> sync_out/1
  sync/1 -> sync_delay/1

== system xblocks_library_downconverter/fir_dbl_col/adder_tree2 ==
  sync : Inport
  din1 : Inport  Port=2
  din2 : Inport  Port=3
  addr1 : xbsIndex_r4/AddSub  mode=Addition  use_carryin=off  use_carryout=off  en=off  latency=1  precision=Full  arith_type=Unsigned  n_bits=16  bin_pt=14  quantization=Truncate  overflow=Wrap  dbl_ovrd=off  use_behavioral_HDL=off  hw_selection=Fabric  pipelined=on  use_rpm=on  block_type=addsub
  sync_delay : xbsIndex_r4/Delay  en=off  latency=1  dbl_ovrd=off  reg_retiming=on  block_type=delay
      settings: block_version=11.4
  sync_out : Outport
  dout : Outport  Port=2
  wires:
  addr1/1 -> dout/1  "adder_outs1_1"
  din2/1 -> addr1/2
  din1/1 -> addr1/1
  sync_delay/1 -> sync_out/1
  sync/1 -> sync_delay/1

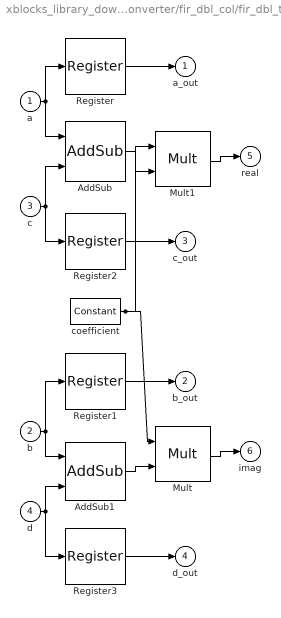
== system xblocks_library_downconverter/fir_dbl_col/fir_dbl_tap1 ==
  a : Inport
  b : Inport  Port=2
  c : Inport  Port=3
  d : Inport  Port=4
  AddSub : xbsIndex_r4/AddSub  mode=Addition  use_carryin=off  use_carryout=off  en=off  latency=1  precision=Full  arith_type="Signed  (2's comp)"  n_bits=18  bin_pt=16  quantization=Truncate  overflow=Wrap  dbl_ovrd=off  use_behavioral_HDL=on  hw_selection=Fabric  pipelined=off  use_rpm=on  block_type=addsub
  AddSub1 : xbsIndex_r4/AddSub  mode=Addition  use_carryin=off  use_carryout=off  en=off  latency=1  precision=Full  arith_type="Signed  (2's comp)"  n_bits=18  bin_pt=16  quantization=Truncate  overflow=Wrap  dbl_ovrd=off  use_behavioral_HDL=on  hw_selection=Fabric  pipelined=off  use_rpm=on  block_type=addsub
  Mult : xbsIndex_r4/Mult  precision=Full  arith_type="Signed  (2's comp)"  n_bits=18  bin_pt=17  quantization=Truncate  overflow=Wrap  en=off  latency=2  dbl_ovrd=off  use_behavioral_HDL=on  opt=Speed  use_embedded=on  optimum_pipeline=off  pipeline=on  use_rpm=off  placement_style=Rectangular shape  block_type=mult
      settings: block_version=11.4
  Mult1 : xbsIndex_r4/Mult  precision=Full  arith_type="Signed  (2's comp)"  n_bits=18  bin_pt=17  quantization=Truncate  overflow=Wrap  en=off  latency=2  dbl_ovrd=off  use_behavioral_HDL=on  opt=Speed  use_embedded=on  optimum_pipeline=off  pipeline=on  use_rpm=off  placement_style=Rectangular shape  block_type=mult
      settings: block_version=11.4
  Register{,1..3} (4 alike) : xbsIndex_r4/Register  init=0  rst=off  en=off  dbl_ovrd=off  block_type=register
      settings: block_version=11.4
  coefficient : xbsIndex_r4/Constant  arith_type=Signed (2's comp)  const=0.1  n_bits=25  bin_pt=24  explicit_period=on  period=1  equ=P=C  opselect=C  inp2=PCIN>>17  opr=+  inp1=P  carry=CIN  dbl_ovrd=off  block_type=constant
      settings: block_version=11.4
  a_out : Outport
  b_out : Outport  Port=2
  c_out : Outport  Port=3
  d_out : Outport  Port=4
  real : Outport  Port=5
  imag : Outport  Port=6
  wires:
  a/1 -> Register/1, AddSub/1
  c/1 -> Register2/1, AddSub/2
  b/1 -> Register1/1, AddSub1/1
  d/1 -> Register3/1, AddSub1/2
  coefficient/1 -> Mult1/1, Mult/1
  Register3/1 -> d_out/1
  Register2/1 -> c_out/1
  Register1/1 -> b_out/1
  Register/1 -> a_out/1
  Mult1/1 -> real/1
  AddSub/1 -> Mult1/2
  Mult/1 -> imag/1
  AddSub1/1 -> Mult/2

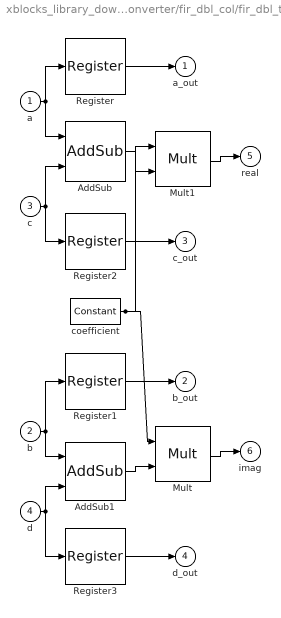
== system xblocks_library_downconverter/fir_dbl_col/fir_dbl_tap2 ==
  a : Inport
  b : Inport  Port=2
  c : Inport  Port=3
  d : Inport  Port=4
  AddSub : xbsIndex_r4/AddSub  mode=Addition  use_carryin=off  use_carryout=off  en=off  latency=1  precision=Full  arith_type="Signed  (2's comp)"  n_bits=18  bin_pt=16  quantization=Truncate  overflow=Wrap  dbl_ovrd=off  use_behavioral_HDL=on  hw_selection=Fabric  pipelined=off  use_rpm=on  block_type=addsub
  AddSub1 : xbsIndex_r4/AddSub  mode=Addition  use_carryin=off  use_carryout=off  en=off  latency=1  precision=Full  arith_type="Signed  (2's comp)"  n_bits=18  bin_pt=16  quantization=Truncate  overflow=Wrap  dbl_ovrd=off  use_behavioral_HDL=on  hw_selection=Fabric  pipelined=off  use_rpm=on  block_type=addsub
  Mult : xbsIndex_r4/Mult  precision=Full  arith_type="Signed  (2's comp)"  n_bits=18  bin_pt=17  quantization=Truncate  overflow=Wrap  en=off  latency=2  dbl_ovrd=off  use_behavioral_HDL=on  opt=Speed  use_embedded=on  optimum_pipeline=off  pipeline=on  use_rpm=off  placement_style=Rectangular shape  block_type=mult
      settings: block_version=11.4
  Mult1 : xbsIndex_r4/Mult  precision=Full  arith_type="Signed  (2's comp)"  n_bits=18  bin_pt=17  quantization=Truncate  overflow=Wrap  en=off  latency=2  dbl_ovrd=off  use_behavioral_HDL=on  opt=Speed  use_embedded=on  optimum_pipeline=off  pipeline=on  use_rpm=off  placement_style=Rectangular shape  block_type=mult
      settings: block_version=11.4
  Register{,1..3} (4 alike) : xbsIndex_r4/Register  init=0  rst=off  en=off  dbl_ovrd=off  block_type=register
      settings: block_version=11.4
  coefficient : xbsIndex_r4/Constant  arith_type=Signed (2's comp)  const=0.2  n_bits=25  bin_pt=24  explicit_period=on  period=1  equ=P=C  opselect=C  inp2=PCIN>>17  opr=+  inp1=P  carry=CIN  dbl_ovrd=off  block_type=constant
      settings: block_version=11.4
  a_out : Outport
  b_out : Outport  Port=2
  c_out : Outport  Port=3
  d_out : Outport  Port=4
  real : Outport  Port=5
  imag : Outport  Port=6
  wires:
  a/1 -> Register/1, AddSub/1
  c/1 -> Register2/1, AddSub/2
  b/1 -> Register1/1, AddSub1/1
  d/1 -> Register3/1, AddSub1/2
  coefficient/1 -> Mult1/1, Mult/1
  Register3/1 -> d_out/1
  Register2/1 -> c_out/1
  Register1/1 -> b_out/1
  Register/1 -> a_out/1
  Mult1/1 -> real/1
  AddSub/1 -> Mult1/2
  Mult/1 -> imag/1
  AddSub1/1 -> Mult/2

== system xblocks_library_downconverter/dec_fir_xblock/fir_col1/adder_tree1 ==
  sync : Inport
  din1 : Inport  Port=2
  din2 : Inport  Port=3
  addr1 : xbsIndex_r4/AddSub  mode=Addition  use_carryin=off  use_carryout=off  en=off  latency=2  precision=Full  arith_type=Unsigned  n_bits=16  bin_pt=14  quantization=Truncate  overflow=Wrap  dbl_ovrd=off  use_behavioral_HDL=off  hw_selection=Fabric  pipelined=on  use_rpm=on  block_type=addsub
  sync_delay : xbsIndex_r4/Delay  rst=off  infoeditControl=Selection of Reset will increase slice count due to use of real FFs and instead of SRLs  en=off  latency=2  dbl_ovrd=off  reg_retiming=on  block_type=delay
  sync_out : Outport
  dout : Outport  Port=2
  wires:
  addr1/1 -> dout/1  "adder_outs1_1"
  din2/1 -> addr1/2
  din1/1 -> addr1/1
  sync_delay/1 -> sync_out/1
  sync/1 -> sync_delay/1

== system xblocks_library_downconverter/dec_fir_xblock/fir_col1/adder_tree2 ==
  sync : Inport
  din1 : Inport  Port=2
  din2 : Inport  Port=3
  addr1 : xbsIndex_r4/AddSub  mode=Addition  use_carryin=off  use_carryout=off  en=off  latency=2  precision=Full  arith_type=Unsigned  n_bits=16  bin_pt=14  quantization=Truncate  overflow=Wrap  dbl_ovrd=off  use_behavioral_HDL=off  hw_selection=Fabric  pipelined=on  use_rpm=on  block_type=addsub
  sync_delay : xbsIndex_r4/Delay  rst=off  infoeditControl=Selection of Reset will increase slice count due to use of real FFs and instead of SRLs  en=off  latency=2  dbl_ovrd=off  reg_retiming=on  block_type=delay
  sync_out : Outport
  dout : Outport  Port=2
  wires:
  addr1/1 -> dout/1  "adder_outs1_1"
  din2/1 -> addr1/2
  din1/1 -> addr1/1
  sync_delay/1 -> sync_out/1
  sync/1 -> sync_delay/1

== system xblocks_library_downconverter/dec_fir_xblock/fir_col1/fir_tap1 ==
  a : Inport
  b : Inport  Port=2
  Constant : xbsIndex_r4/Constant  const=2  gui_display_data_type=Fixed-point  arith_type=Signed (2's comp)  n_bits=25  bin_pt=24  preci_type=Single  exp_width=8  frac_width=24  explicit_period=on  period=1  equ=P=C  opselect=C  inp2=PCIN>>17  opr=+  inp1=P  carry=CIN  dbl_ovrd=off  block_type=constant
  Mult : xbsIndex_r4/Mult  precision=Full  arith_type="Signed  (2's comp)"  n_bits=18  bin_pt=17  quantization=Truncate  overflow=Wrap  en=off  latency=1  dbl_ovrd=off  use_behavioral_HDL=on  opt=Speed  use_embedded=on  optimum_pipeline=off  pipeline=on  use_rpm=off  placement_style=Rectangular shape  block_type=mult
  Mult1 : xbsIndex_r4/Mult  precision=Full  arith_type="Signed  (2's comp)"  n_bits=18  bin_pt=17  quantization=Truncate  overflow=Wrap  en=off  latency=1  dbl_ovrd=off  use_behavioral_HDL=on  opt=Speed  use_embedded=on  optimum_pipeline=off  pipeline=on  use_rpm=off  placement_style=Rectangular shape  block_type=mult
  Register : xbsIndex_r4/Register  init=0  rst=off  en=off  dbl_ovrd=off  block_type=register
  Register1 : xbsIndex_r4/Register  init=0  rst=off  en=off  dbl_ovrd=off  block_type=register
  a_out : Outport
  b_out : Outport  Port=2
  real : Outport  Port=3
  imag : Outport  Port=4
  wires:
  Constant/1 -> Mult1/1, Mult/1
  b/1 -> Register1/1, Mult/2
  a/1 -> Register/1, Mult1/2
  Register1/1 -> b_out/1
  Register/1 -> a_out/1
  Mult1/1 -> real/1
  Mult/1 -> imag/1

== system xblocks_library_downconverter/dec_fir_xblock/fir_col1/fir_tap2 ==
  a : Inport
  b : Inport  Port=2
  Constant : xbsIndex_r4/Constant  const=1  gui_display_data_type=Fixed-point  arith_type=Signed (2's comp)  n_bits=25  bin_pt=24  preci_type=Single  exp_width=8  frac_width=24  explicit_period=on  period=1  equ=P=C  opselect=C  inp2=PCIN>>17  opr=+  inp1=P  carry=CIN  dbl_ovrd=off  block_type=constant
  Mult : xbsIndex_r4/Mult  precision=Full  arith_type="Signed  (2's comp)"  n_bits=18  bin_pt=17  quantization=Truncate  overflow=Wrap  en=off  latency=1  dbl_ovrd=off  use_behavioral_HDL=on  opt=Speed  use_embedded=on  optimum_pipeline=off  pipeline=on  use_rpm=off  placement_style=Rectangular shape  block_type=mult
  Mult1 : xbsIndex_r4/Mult  precision=Full  arith_type="Signed  (2's comp)"  n_bits=18  bin_pt=17  quantization=Truncate  overflow=Wrap  en=off  latency=1  dbl_ovrd=off  use_behavioral_HDL=on  opt=Speed  use_embedded=on  optimum_pipeline=off  pipeline=on  use_rpm=off  placement_style=Rectangular shape  block_type=mult
  Register : xbsIndex_r4/Register  init=0  rst=off  en=off  dbl_ovrd=off  block_type=register
  Register1 : xbsIndex_r4/Register  init=0  rst=off  en=off  dbl_ovrd=off  block_type=register
  a_out : Outport
  b_out : Outport  Port=2
  real : Outport  Port=3
  imag : Outport  Port=4
  wires:
  Constant/1 -> Mult1/1, Mult/1
  b/1 -> Register1/1, Mult/2
  a/1 -> Register/1, Mult1/2
  Register1/1 -> b_out/1
  Register/1 -> a_out/1
  Mult1/1 -> real/1
  Mult/1 -> imag/1

== system xblocks_library_downconverter/dec_fir_xblock/fir_col2/adder_tree1 ==
  sync : Inport
  din1 : Inport  Port=2
  din2 : Inport  Port=3
  addr1 : xbsIndex_r4/AddSub  mode=Addition  use_carryin=off  use_carryout=off  en=off  latency=2  precision=Full  arith_type=Unsigned  n_bits=16  bin_pt=14  quantization=Truncate  overflow=Wrap  dbl_ovrd=off  use_behavioral_HDL=off  hw_selection=Fabric  pipelined=on  use_rpm=on  block_type=addsub
  sync_delay : xbsIndex_r4/Delay  rst=off  infoeditControl=Selection of Reset will increase slice count due to use of real FFs and instead of SRLs  en=off  latency=2  dbl_ovrd=off  reg_retiming=on  block_type=delay
  sync_out : Outport
  dout : Outport  Port=2
  wires:
  addr1/1 -> dout/1  "adder_outs1_1"
  din2/1 -> addr1/2
  din1/1 -> addr1/1
  sync_delay/1 -> sync_out/1
  sync/1 -> sync_delay/1

== system xblocks_library_downconverter/dec_fir_xblock/fir_col2/adder_tree2 ==
  sync : Inport
  din1 : Inport  Port=2
  din2 : Inport  Port=3
  addr1 : xbsIndex_r4/AddSub  mode=Addition  use_carryin=off  use_carryout=off  en=off  latency=2  precision=Full  arith_type=Unsigned  n_bits=16  bin_pt=14  quantization=Truncate  overflow=Wrap  dbl_ovrd=off  use_behavioral_HDL=off  hw_selection=Fabric  pipelined=on  use_rpm=on  block_type=addsub
  sync_delay : xbsIndex_r4/Delay  rst=off  infoeditControl=Selection of Reset will increase slice count due to use of real FFs and instead of SRLs  en=off  latency=2  dbl_ovrd=off  reg_retiming=on  block_type=delay
  sync_out : Outport
  dout : Outport  Port=2
  wires:
  addr1/1 -> dout/1  "adder_outs1_1"
  din2/1 -> addr1/2
  din1/1 -> addr1/1
  sync_delay/1 -> sync_out/1
  sync/1 -> sync_delay/1

== system xblocks_library_downconverter/dec_fir_xblock/fir_col2/fir_tap1 ==
  a : Inport
  b : Inport  Port=2
  Constant : xbsIndex_r4/Constant  const=4  gui_display_data_type=Fixed-point  arith_type=Signed (2's comp)  n_bits=25  bin_pt=24  preci_type=Single  exp_width=8  frac_width=24  explicit_period=on  period=1  equ=P=C  opselect=C  inp2=PCIN>>17  opr=+  inp1=P  carry=CIN  dbl_ovrd=off  block_type=constant
  Mult : xbsIndex_r4/Mult  precision=Full  arith_type="Signed  (2's comp)"  n_bits=18  bin_pt=17  quantization=Truncate  overflow=Wrap  en=off  latency=1  dbl_ovrd=off  use_behavioral_HDL=on  opt=Speed  use_embedded=on  optimum_pipeline=off  pipeline=on  use_rpm=off  placement_style=Rectangular shape  block_type=mult
  Mult1 : xbsIndex_r4/Mult  precision=Full  arith_type="Signed  (2's comp)"  n_bits=18  bin_pt=17  quantization=Truncate  overflow=Wrap  en=off  latency=1  dbl_ovrd=off  use_behavioral_HDL=on  opt=Speed  use_embedded=on  optimum_pipeline=off  pipeline=on  use_rpm=off  placement_style=Rectangular shape  block_type=mult
  Register : xbsIndex_r4/Register  init=0  rst=off  en=off  dbl_ovrd=off  block_type=register
  Register1 : xbsIndex_r4/Register  init=0  rst=off  en=off  dbl_ovrd=off  block_type=register
  a_out : Outport
  b_out : Outport  Port=2
  real : Outport  Port=3
  imag : Outport  Port=4
  wires:
  Constant/1 -> Mult1/1, Mult/1
  b/1 -> Register1/1, Mult/2
  a/1 -> Register/1, Mult1/2
  Register1/1 -> b_out/1
  Register/1 -> a_out/1
  Mult1/1 -> real/1
  Mult/1 -> imag/1

== system xblocks_library_downconverter/dec_fir_xblock/fir_col2/fir_tap2 ==
  a : Inport
  b : Inport  Port=2
  Constant : xbsIndex_r4/Constant  const=3  gui_display_data_type=Fixed-point  arith_type=Signed (2's comp)  n_bits=25  bin_pt=24  preci_type=Single  exp_width=8  frac_width=24  explicit_period=on  period=1  equ=P=C  opselect=C  inp2=PCIN>>17  opr=+  inp1=P  carry=CIN  dbl_ovrd=off  block_type=constant
  Mult : xbsIndex_r4/Mult  precision=Full  arith_type="Signed  (2's comp)"  n_bits=18  bin_pt=17  quantization=Truncate  overflow=Wrap  en=off  latency=1  dbl_ovrd=off  use_behavioral_HDL=on  opt=Speed  use_embedded=on  optimum_pipeline=off  pipeline=on  use_rpm=off  placement_style=Rectangular shape  block_type=mult
  Mult1 : xbsIndex_r4/Mult  precision=Full  arith_type="Signed  (2's comp)"  n_bits=18  bin_pt=17  quantization=Truncate  overflow=Wrap  en=off  latency=1  dbl_ovrd=off  use_behavioral_HDL=on  opt=Speed  use_embedded=on  optimum_pipeline=off  pipeline=on  use_rpm=off  placement_style=Rectangular shape  block_type=mult
  Register : xbsIndex_r4/Register  init=0  rst=off  en=off  dbl_ovrd=off  block_type=register
  Register1 : xbsIndex_r4/Register  init=0  rst=off  en=off  dbl_ovrd=off  block_type=register
  a_out : Outport
  b_out : Outport  Port=2
  real : Outport  Port=3
  imag : Outport  Port=4
  wires:
  Constant/1 -> Mult1/1, Mult/1
  b/1 -> Register1/1, Mult/2
  a/1 -> Register/1, Mult1/2
  Register1/1 -> b_out/1
  Register/1 -> a_out/1
  Mult1/1 -> real/1
  Mult/1 -> imag/1
